simulink model "zadacha_16_03"  (Simulink 7.1)
settings: Solver=ode45  StartTime=0.0  StopTime=100  RelTol=1e-3
settings Model: Creator=Slavi  LastModifiedBy=Slavi

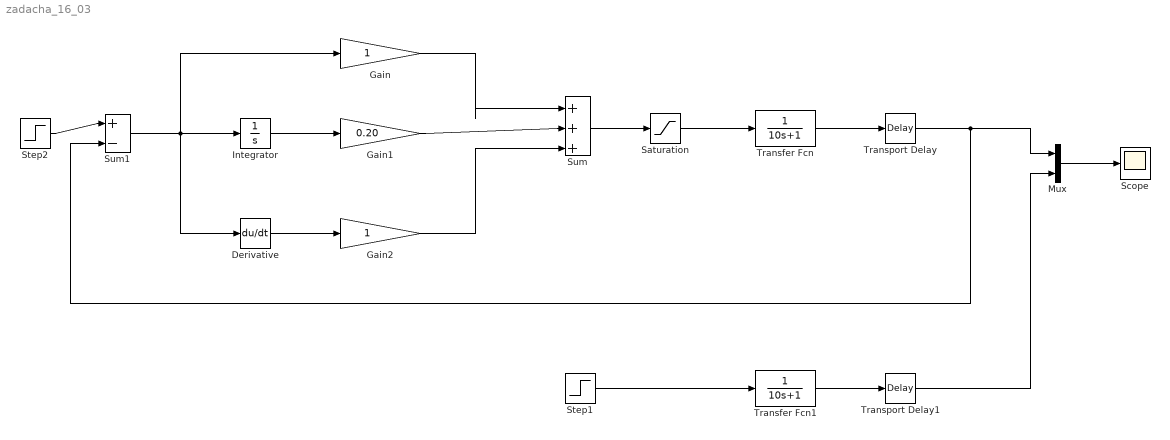
== system zadacha_16_03 ==
  Derivative : Derivative
  Gain : Gain  ParameterDataType=sfix(16)  ParameterScaling=2^0  OutDataType=sfix(16)  OutScaling=2^0
  Gain1 : Gain  Gain=0.20  ParameterDataType=sfix(16)  ParameterScaling=2^0  OutDataType=sfix(16)  OutScaling=2^0
  Gain2 : Gain  ParameterDataType=sfix(16)  ParameterScaling=2^0  OutDataType=sfix(16)  OutScaling=2^0
  Integrator : Integrator
  Mux : Mux  Inputs=2
  Saturation : Saturate  UpperLimit=10  LowerLimit=-10  OutDataType=sfix(16)  OutScaling=2^0
  Scope : Scope
  Step1 : Step
  Step2 : Step
  Sum : Sum  Inputs=|+++  OutDataType=sfix(16)  OutScaling=2^0
  Sum1 : Sum  Inputs=|+-  OutDataType=sfix(16)  OutScaling=2^0
  Transfer Fcn : TransferFcn  Denominator=[10 1]
  Transfer Fcn1 : TransferFcn  Denominator=[10 1]
  Transport Delay : TransportDelay  DelayTime=2
  Transport Delay1 : TransportDelay  DelayTime=2
  wires:
  Mux/1 -> Scope/1
  Transfer Fcn/1 -> Transport Delay/1
  Transport Delay/1 -> Mux/1, Sum1/2
  Step1/1 -> Transfer Fcn1/1
  Transfer Fcn1/1 -> Transport Delay1/1
  Transport Delay1/1 -> Mux/2
  Integrator/1 -> Gain1/1
  Derivative/1 -> Gain2/1
  Gain1/1 -> Sum/2
  Gain2/1 -> Sum/3
  Gain/1 -> Sum/1
  Sum1/1 -> Gain/1, Derivative/1, Integrator/1
  Sum/1 -> Saturation/1
  Step2/1 -> Sum1/1
  Saturation/1 -> Transfer Fcn/1
